simulink model "AGI_hydrogen_test9"  (R2024b)
settings: Solver=VariableStepAuto  StartTime=0.0  StopTime=Test.t_sim  RelTol=1e-3
values from neighbouring files (symbols this model uses):
  ControlSampleTime = 1/8000    (= 0.000125)    [init.m]
  f_Batt_ref = [46 47 49.9 50.1 52 53]    [init.m]
  f_PV_ref = [46 50.1 52 53]    [init.m]
  Hy_current_Ki = 20    [init.m]
  Hy_current_Kp = 0.3    [init.m]
  P_Batt_ref = [0.5 0.5 0 0 -0.5 -0.5]    [init.m]
  P_PV_ref = [1 1 1 1]    [init.m]
  PLL_Ki = 100    [init.m]
  PLL_Kp = 30    [init.m]
  Q_Batt_ref = [-0.5 -0.5 0 0.5 0.5]    [init.m]
  Q_PV_ref = [-0.5 -0.5 0 0.5 0.5]    [init.m]
  Q_ref_pu_VSM = 1    [init.m]
  S_AGI = SC_AGI    (= 25000)    [init.m]
  Test =     [S-Rocof1-OC1.mat]    (also in S-VolAngStep4-OC1.mat)
  Ts = ControlSampleTime    (= 0.000125)    [init.m]
  Ts_Control = 1e-4    (= 0.0001)    [init.m]
  Ts_Power = 5e-5    (= 5e-05)    [init.m]
  U_Batt_ref = [0.8 0.9 1 1.1 1.2]    [init.m]
  U_PV_ref = [0.8 0.9 1 1.1 1.2]    [init.m]
undefined symbols (not defined in the file or in its folder): DiscIntNeverNeededParam, Grid, Ion, L_line_PV, LCL, Lithium, sps, VSMCTRL
libraries: spsThreePhaseSeriesRLCBranchLib x10, powerlib_extras x9, spsSeriesRLCBranchLib x8, spsThreePhaseVIMeasurementLib x6, spsThreePhaseBreakerLib x6, slpidlib x6, simulink x6, spsVoltageMeasurementLib x6, FriedrichLibrary x6, spsPowerPositiveSequenceLib x5, spsUniversalBridgeLib x4, spsControlledVoltageSourceLib x4
(part 3 of 3)

== system AGI_hydrogen_test9/PV/VSC Control1/VDC Regulator ==
  Vdc_meas : Inport  PortDimensions=1
  Vdc_ref : Inport  Port=2  PortDimensions=1
  PI : slpidlib/PID Controller  Controller=PI  Form=Parallel  TimeDomain=Discrete-time  UseExternalTs=off  SampleTime=Ts  IntegratorMethod=Trapezoidal  FilterMethod=Forward Euler  ControllerParametersSource=internal  P=Kp_VDCreg  I=Ki_VDCreg  UseKiTs=off  D=0  UseExternalDerivativeSource=off  N=100  UseFilter=on  TunerSelectOption=Transfer Function Based (PID Tuner App)  InitialConditionSource=internal  InitialConditionForIntegrator=0  InitialConditionForFilter=0  DifferentiatorICPrevScaledInput=0  ExternalReset=none  TrackingMode=off  Kt=1  LimitOutput=on  SatLimitsSource=internal  UpperSaturationLimit=1.5  LowerSaturationLimit=-1.5  LinearizeAsGain=off  AntiWindupMode=back-calculation  Kb=Ki_VDCreg  LimitIntegrator=on  UpperIntegratorSaturationLimit=1.5  LowerIntegratorSaturationLimit=-inf  POutMin=[]  POutMax=[]  IOutMin=[]  IOutMax=[]  DOutMin=[]  DOutMax=[]  NOutMin=[]  NOutMax=[]  SumOutMin=[]  SumOutMax=[]  SaturationOutMin=[]  SaturationOutMax=[]  PParamMin=[]  PParamMax=[]  IParamMin=[]  IParamMax=[]  DParamMin=[]  DParamMax=[]  NParamMin=[]  NParamMax=[]  KbParamMin=[]  KbParamMax=[]  KtParamMin=[]  KtParamMax=[]  KbOutMin=[]  KbOutMax=[]  KtOutMin=[]  KtOutMax=[]  IntegratorOutMin=[]  IntegratorOutMax=[]  FilterOutMin=[]  FilterOutMax=[]  SumI1OutMin=[]  SumI1OutMax=[]  SumI2OutMin=[]  SumI2OutMax=[]  SumI3OutMin=[]  SumI3OutMax=[]  SumI4OutMin=[]  SumI4OutMax=[]  SumDOutMin=[]  SumDOutMax=[]  DifferentiatorOutMin=[]  DifferentiatorOutMax=[]  FilterDiffOutCoefMin=[]  FilterDiffOutCoefMax=[]  ReciprocalOutMin=[]  ReciprocalOutMax=[]  SumDenOutMin=[]  SumDenOutMax=[]  SumNumOutMin=[]  SumNumOutMax=[]  DivideOutMin=[]  DivideOutMax=[]  UdiffTsProdOutMin=[]  UdiffTsProdOutMax=[]  NTsProdOutMin=[]  NTsProdOutMax=[]  UintegralTsProdOutMin=[]  UintegralTsProdOutMax=[]  UngainTsProdOutMin=[]  UngainTsProdOutMax=[]  ClampingZeroOutDataTypeStr=Inherit: Inherit via back propagation  ClampingZeroOutMin=[]  ClampingZeroOutMax=[]  FilterDenConstantOutDataTypeStr=Inherit: Inherit via back propagation  FilterDenConstantOutMin=[]  FilterDenConstantOutMax=[]  PCopyOutDataTypeStr=Inherit: Inherit via back propagation  PCopyOutMin=[]  PCopyOutMax=[]  NCopyOutDataTypeStr=Inherit: Inherit via back propagation  NCopyOutMin=[]  NCopyOutMax=[]  IntegratorContinuousStateAttributes=''  IntegratorStateMustResolveToSignalObject=off  IntegratorRTWStateStorageClass=Auto  FilterContinuousStateAttributes=''  FilterStateMustResolveToSignalObject=off  FilterRTWStateStorageClass=Auto  ParallelPVariant=InternalParameters  IdealPVariant=Disabled  IVariant=InternalParameters  DVariant=Disabled  IntegratorVariant=Discrete  SatVariant=Enabled  AWVariant=BackCalculation  PCopyVariant=Disabled  TRVariant=Disabled  FdbkBlocksVariant=Feedback  IdealPFdbkVariant=Passthrough  SatFdbkVariant=Enabled  DerivativeFilterVariant=Disabled  NVariant=Disabled  NCopyVariant=Disabled_SignalSpec  FilterICVariant=Disabled  IntegratorICVariant=InternalICs  ExternalResetVariant=Disabled  TRSumVariant=Passthrough  SumFdbkVariant=Enabled  SumVariant=Sum_PI  TsampFilterVariant=InternalTs  TsampNgainVariant=Passthrough  TsampIntegralVariant=Disabled_SignalSpec  ExternalSaturationOutDataTypeStr=Inherit: Same as second input  DerivativeSourceVariant=Disabled  PreIntVariant=InternalPreInt
  Rtot_pu3 : Gain  Gain=1/Vnom_dc  SaturateOnIntegerOverflow=on  OutDataTypeStr=Inherit: Same as input  ParamDataTypeStr=Inherit: Same as input
  Sum : Sum  Inputs=|+-
  Id_ref : Outport  SampleTime=Ts  InitialOutput=0  VectorParamsAs1DForOutWhenUnconnected=off
  wires:
  PI/1 -> Id_ref/1, [Id_ref]
  Rtot_pu3/1 -> PI/1
  Vdc_ref/1 -> [Vdc_ref], Sum/2
  Vdc_meas/1 -> Sum/1
  Sum/1 -> Rtot_pu3/1

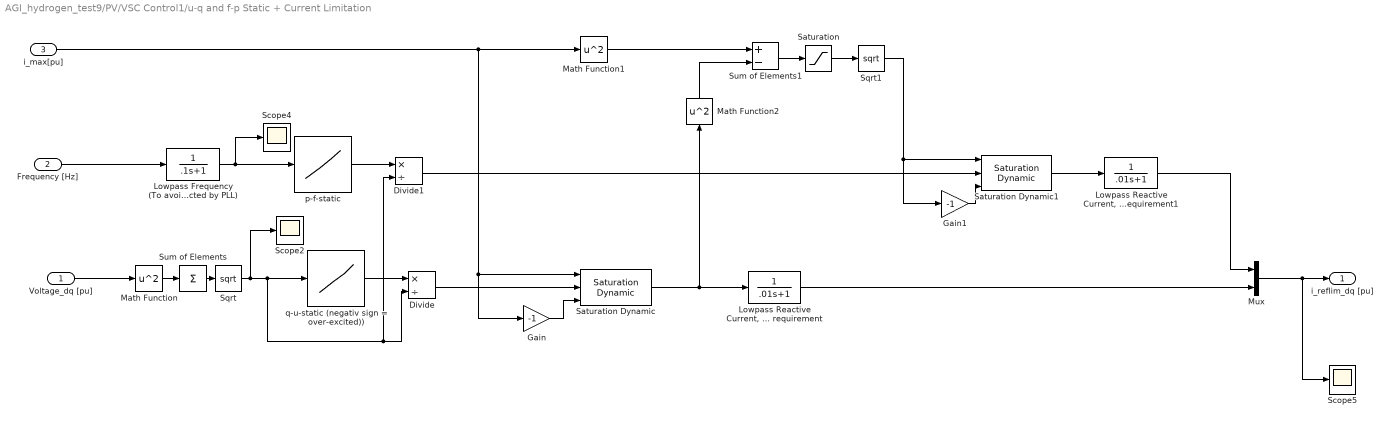
== system AGI_hydrogen_test9/PV/VSC Control1/u-q and f-p Static + Current Limitation ==
  Voltage_dq [pu] : Inport
  Frequency [Hz] : Inport  Port=2
  i_max[pu] : Inport  Port=3
  Divide : Product  Inputs=*/
  Divide1 : Product  Inputs=*/
  Gain : Gain  Gain=-1
  Gain1 : Gain  Gain=-1
  Lowpass Frequency (To avoid unstable Interaction with PLL because change in P will change phase angle which is detected by PLL) : TransferFcn  Denominator=[.1 1]
  "Lowpass Reactive Current, see grid code for dynamic requirement" : TransferFcn  Denominator=[.01 1]
  "Lowpass Reactive Current, see grid code for dynamic requirement1" : TransferFcn  Denominator=[.01 1]
  Math Function : Math  Operator=square
  Math Function1 : Math  Operator=square
  Math Function2 : Math  Operator=square
  Mux : Mux  Inputs=2
  Saturation : Saturate  UpperLimit=inf  LowerLimit=0
  Saturation Dynamic : simulink/Discontinuities/Saturation Dynamic  OutMin=[]  OutMax=[]  OutDataTypeStr=Inherit: Same as second input  OutDataType=fixdt(1, 16)  OutScaling=2^-10  DoSatur=off
  Saturation Dynamic1 : simulink/Discontinuities/Saturation Dynamic  OutMin=[]  OutMax=[]  OutDataTypeStr=Inherit: Same as second input  OutDataType=fixdt(1, 16)  OutScaling=2^-10  DoSatur=off
  Scope2 : Scope
  Scope4 : Scope
  Scope5 : Scope
  Sqrt : Sqrt
  Sqrt1 : Sqrt
  Sum of Elements : Sum  Inputs=+
  Sum of Elements1 : Sum  Inputs=+-
  "p-f-static " : Lookup_n-D  NumberOfTableDimensions=1  BreakpointsForDimension1=f_PV_ref  Table=P_PV_ref  InternalRulePriority=Speed  RndMeth=Simplest
  q-u-static (negativ sign = over-excited)) : Lookup_n-D  NumberOfTableDimensions=1  BreakpointsForDimension1=U_PV_ref  Table=Q_PV_ref  InternalRulePriority=Speed  RndMeth=Simplest
  i_reflim_dq [pu] : Outport
  wires:
  Sqrt/1 -> Scope2/1, q-u-static (negativ sign = over-excited))/1, Divide/2, Divide1/2
  Sum of Elements/1 -> Sqrt/1
  Math Function/1 -> Sum of Elements/1
  "p-f-static "/1 -> Divide1/1
  Frequency [Hz]/1 -> Lowpass Frequency (To avoid unstable Interaction with PLL because change in P will change phase angle which is detected by PLL)/1
  Lowpass Frequency (To avoid unstable Interaction with PLL because change in P will change phase angle which is detected by PLL)/1 -> Scope4/1, "p-f-static "/1
  q-u-static (negativ sign = over-excited))/1 -> Divide/1
  Divide/1 -> Saturation Dynamic/2
  Voltage_dq [pu]/1 -> Math Function/1
  Mux/1 -> Scope5/1, i_reflim_dq [pu]/1
  Divide1/1 -> Saturation Dynamic1/2
  Saturation Dynamic/1 -> "Lowpass Reactive Current, see grid code for dynamic requirement"/1, Math Function2/1
  i_max[pu]/1 -> Math Function1/1, Saturation Dynamic/1, Gain/1
  Math Function1/1 -> Sum of Elements1/1
  Math Function2/1 -> Sum of Elements1/2
  Sum of Elements1/1 -> Saturation/1
  Saturation/1 -> Sqrt1/1
  Sqrt1/1 -> Saturation Dynamic1/1, Gain1/1
  Saturation Dynamic1/1 -> "Lowpass Reactive Current, see grid code for dynamic requirement1"/1
  Gain/1 -> Saturation Dynamic/3
  Gain1/1 -> Saturation Dynamic1/3
  "Lowpass Reactive Current, see grid code for dynamic requirement"/1 -> Mux/2
  "Lowpass Reactive Current, see grid code for dynamic requirement1"/1 -> Mux/1

== system AGI_hydrogen_test9/VSM with SC/VSM1/Integrator (Angle) ==
  Reset : Inport
  omega : Inport  Port=2
  d_phi0 : Inport  Port=3
  Angle Integrator Reset[SI] : FriedrichLibrary/Discrete Stuff/Angle Integrator Reset[SI]  Ts=ControlSampleTime
  Delay : Delay  DelayLength=1  InitialConditionSource=Input port
      settings: InputPortMap=u0,p4
  Gain3 : Gain  Gain=-1*ControlSampleTime
  Scope : Scope  NumInputPorts=2
  Scope1 : Scope  NumInputPorts=2
  Sum1 : Sum  Inputs=|++
  Sum9 : Sum  Inputs=|+-
  phi : Outport  VectorParamsAs1DForOutWhenUnconnected=off
  wires:
  Gain3/1 -> Sum9/2, Scope/2, Delay/2
  omega/1 -> Gain3/1, Angle Integrator Reset[SI]/2
  Angle Integrator Reset[SI]/1 -> Delay/1, phi/1  "Phi [rad]"
  Reset/1 -> Scope1/1, Angle Integrator Reset[SI]/1
  Sum9/1 -> Sum1/1
  Sum1/1 -> Scope1/2, Angle Integrator Reset[SI]/3
  d_phi0/1 -> Sum9/1
  Delay/1 -> Scope/1, Sum1/2

== system AGI_hydrogen_test9/VSM with SC/VSM1/Integrator (Inertia) ==
  dPTa : Inport
  omega0 [pu] : Inport  Port=2
  Enable : EnablePort
  Integrator (inertia) : DiscreteIntegrator  gainval=1  InitialConditionSource=external  InitialCondition=1  SampleTime=ControlSampleTime  ICPrevOutput=DiscIntNeverNeededParam  ICPrevScaledInput=DiscIntNeverNeededParam
  omega [pu] : Outport  VectorParamsAs1DForOutWhenUnconnected=off
  wires:
  omega0 [pu]/1 -> Integrator (inertia)/2
  Integrator (inertia)/1 -> omega [pu]/1  "Omega [pu]"
  dPTa/1 -> Integrator (inertia)/1

== system AGI_hydrogen_test9/PV/DC//DC 1/Boost Converter (Average Model)/Prediction ==
  In : Inport
  Gain : Gain  Gain=2
  Subtract2 : Sum  Inputs=+-
  prediction : UnitDelay  SampleTime=Ts  HasFrameUpgradeWarning=on
  Out : Outport  VectorParamsAs1DForOutWhenUnconnected=off
  wires:
  prediction/1 -> Subtract2/2
  In/1 -> prediction/1, Gain/1
  Subtract2/1 -> Out/1
  Gain/1 -> Subtract2/1

== system AGI_hydrogen_test9/PV/DC//DC 1/Boost Converter (Average Model)/scaling1 ==
  note: Shifting from ]0 to 1[ to a ]-1 to 1[ scale
  D : Inport
  Bias : Bias  Bias=-0.5  SaturateOnIntegerOverflow=off
  Gain : Gain  Gain=2
  Saturation : Saturate  UpperLimit=1  LowerLimit=-1
  m : Outport  VectorParamsAs1DForOutWhenUnconnected=off
  wires:
  Saturation/1 -> m/1
  Gain/1 -> Saturation/1
  D/1 -> Bias/1
  Bias/1 -> Gain/1

== matlab function AGI_hydrogen_test9/PV/DC//DC 1/MPPT Control   ==
  settings: updateMethod=DISCRETE  sampleTime=Ts_Control
  data: Param input; Enabled input; V input =V; I input; D output
function D  = PandO(Param, Enabled, V, I)

% MPPT controller based on the Perturb & Observe algorithm.

% D output = Duty cycle of the boost converter (value between 0 and 1)
%
% Enabled input = 1 to enable the MPPT controller
% V input = PV array terminal voltage (V)
% I input = PV array current (A)
%
% Param input:
Dinit = Param(1);  %Initial value for D output
Dmax = Param(2);   %Maximum value for D
Dmin = Param(3);   %Minimum value for D
deltaD = Param(4); %Increment value used to increase/decrease the duty cycle D
% ( increasing D = decreasing Vref )
%  

persistent Vold Pold Dold;

dataType = 'double';

if isempty(Vold)
    Vold=0;
    Pold=0;
    Dold=Dinit;
end
P= V*I;
dV= V - Vold;
dP= P - Pold;

if dP ~= 0 & Enabled ~=0
    if dP < 0
        if dV < 0
            D = Dold - deltaD;
        else
            D = Dold + deltaD;
        end
    else
        if dV < 0
            D = Dold + deltaD;
        else
            D = Dold - deltaD;
        end    
    end
else D=Dold;
end

if D >= Dmax | D<= Dmin
    D=Dold;
end

Dold=D;
Vold=V;
Pold=P;
